simulink model "mod_serbatoi"  (Simulink 7.6)
settings: Solver=ode45  StartTime=0.0  StopTime=10.0  MaxStep=.01  RelTol=1e-3
values from neighbouring files (symbols this model uses):
  A = [0 1;-k/m -b/m]    [massamollasmorz.m]    (also in serbatoi.m = [ -k1/S1 0; k1/S2 -k2/S2 ])
  B = [0;1/m]    [massamollasmorz.m]    (also in serbatoi.m = [ 1/S1; 0 ])
  ueq = 2    [massamollasmorz.m]    (also in serbatoi.m = 1)
libraries: simulink x1
settings Model: Creator=patrizio  LastModifiedBy=patrizio

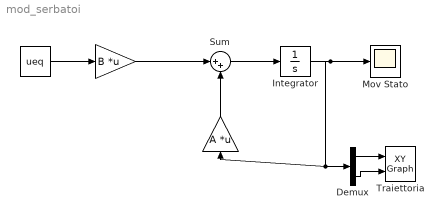
== system mod_serbatoi ==
  " " : Gain  Gain=B  Multiplication=Matrix(K*u)
  "  " : Gain  Gain=A  Multiplication=Matrix(K*u)
  "   " : Constant  Value=ueq
  Demux : Demux  Outputs=2
  Integrator : Integrator
  Mov Stato : Scope
      settings: TimeRange=10  YMin=0  YMax=2
  Sum : Sum  Inputs=|++
  Traiettoria : simulink/Sinks/XY Graph  SystemSampleTime=-1  xmin=0  xmax=10  ymin=0  ymax=2  st=-1
  wires:
  "   "/1 -> " "/1
  " "/1 -> Sum/1
  Sum/1 -> Integrator/1
  Integrator/1 -> Mov Stato/1, "  "/1, Demux/1
  "  "/1 -> Sum/2
  Demux/2 -> Traiettoria/2
  Demux/1 -> Traiettoria/1
